simulink subsystem "heat_sink"  (R2020b)
settings: Solver=VariableStepAuto  StartTime=0.0  StopTime=10.0  RelTol=1e-3
model mask{fidelityPARAM=Reduced Order Model, freqPARAM=[-Inf 20], kPARAM=64}
  mask prompts: fidelityPARAM "Choose fidelity:"; freqPARAM "Frequency Range:"; kPARAM "Frequencies retained:"
values from neighbouring files (symbols this model uses):
  h_forced = [  0.0, h_free;  3.0, 50.0;  ]    [heat_sink_defs.m]
  h_free = 9.0    (= 9)    [heat_sink_defs.m]
  normalizedForcedBC = zeros(nDoF,1)    [heat_sink_defs.m]
  normalizedFreeBC = zeros(nDoF,1)    [heat_sink_defs.m]
  Tinf = IC    (= 294)    [heat_sink_defs.m]
  unitCPUHeat = full(F)    [heat_sink_defs.m]
  unitForcedBC = zeros(nDoF,1)    [heat_sink_defs.m]
  unitFreeBC = zeros(nDoF,1)    [heat_sink_defs.m]
  x0 = ones(nDoF,1)*IC    [heat_sink_defs.m]
undefined symbols (not defined in the file or in its folder): Ar, Br, Cr, Dr, sparse, speye, V
settings Model: Creator=jclinton  LastModifiedBy=jclinton
settings DebuggingCC: SFMachineParentedDataDiag=error

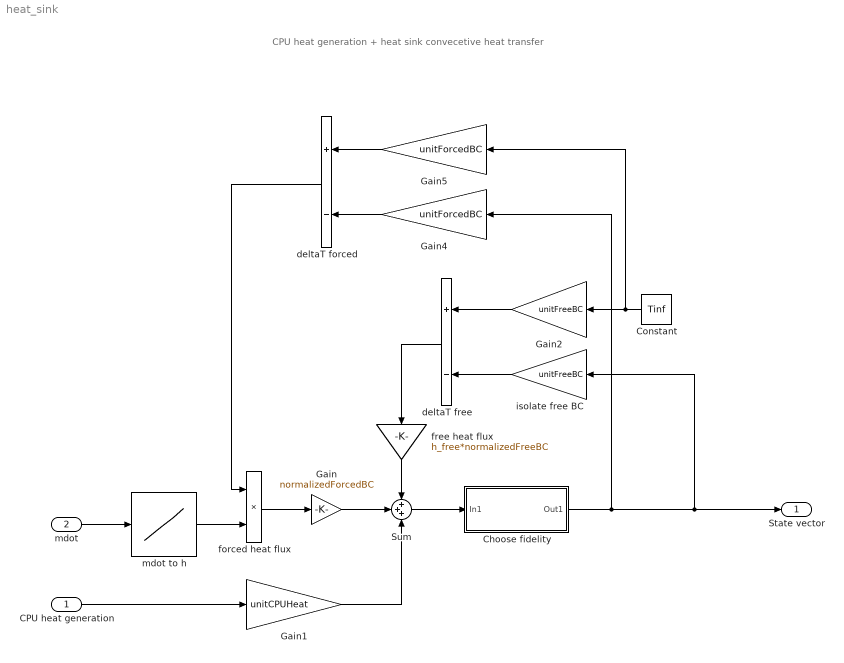
== system heat_sink ==
  note: CPU heat generation + heat sink convecetive heat transfer
  CPU heat generation : Inport  Unit=W
  mdot : Inport  Port=2  Unit=kg/sec
  Choose fidelity : Subsystem  Variant=on  VariantControlMode=label  LabelModeActiveChoice=Choice_2
      mask init:
      | fidelity = get_param(gcs,'fidelityPARAM');
      | vssBlk = gcb;
      | if strcmp(fidelity,'Finite Element Model')
      |     set_param(vssBlk, 'LabelModeActiveChoice', 'Choice_1');
      | else
      |     set_param(vssBlk, 'LabelModeActiveChoice', 'Choice_2');
      |     Q = evalin('base','Q');
      |     K = evalin('base','K');
      |     nDoF = evalin('base','nDoF');
      |     M = evalin('base','M');
      |     freq = str2num(get_param(gcs,'freqPARAM'));
      |     k = str2num(get_param(gcs,'kPARAM'));
      |     [Ar,Br,Cr,Dr,Er,V] = reduceModelOrder(Q+K, ...
      |                                           speye(nDoF,nDoF), ...
      |                                           speye(nDoF,nDoF), ...
      |                                           sparse(nDoF,nDoF), ...
      |                                           M, ...
      |                                           freq,...
      |                                           k);
      | end
      mask DialogControl DescGroupVar Prompt: Choose between FE formulation or a reduced order model
      mask DialogControl DescTextVar Prompt: Different DSS blocks underneath mask chosen depending on desirede fidelity
      mask Display: disp('\partialu/\partialt = \alpha(\Deltau)','texmode','on')
  Constant : Constant  Value=Tinf
  Gain : Gain  Gain=normalizedForcedBC
  Gain1 : Gain  Gain=unitCPUHeat
  Gain2 : Gain  Gain=unitFreeBC
  Gain4 : Gain  Gain=unitForcedBC
  Gain5 : Gain  Gain=unitForcedBC
  Sum : Sum  Inputs=+++
  "deltaT forced " : Sum  Inputs=+-
  deltaT free : Sum  Inputs=+-
  forced heat flux : Product
  free heat flux : Gain  Gain=h_free*normalizedFreeBC
  isolate free BC : Gain  Gain=unitFreeBC
  mdot to h : Lookup_n-D  NumberOfTableDimensions=1  BreakpointsForDimension1=h_forced(:,1)  Table=h_forced(:,2)  InternalRulePriority=Speed  RndMeth=Simplest  InputSameDT=on
  State vector : Outport  Unit=K
  wires:
  mdot/1 -> mdot to h/1
  mdot to h/1 -> forced heat flux/2
  forced heat flux/1 -> Gain/1
  Gain/1 -> Sum/2
  free heat flux/1 -> Sum/1
  deltaT free/1 -> free heat flux/1
  Gain2/1 -> deltaT free/1
  Constant/1 -> Gain5/1, Gain2/1
  isolate free BC/1 -> deltaT free/2
  Gain4/1 -> "deltaT forced "/2
  Gain5/1 -> "deltaT forced "/1
  "deltaT forced "/1 -> forced heat flux/1
  CPU heat generation/1 -> Gain1/1
  Gain1/1 -> Sum/3
  Choose fidelity/1(Out1) -> Gain4/1, State vector/1, isolate free BC/1
  Sum/1 -> Choose fidelity/1(In1)

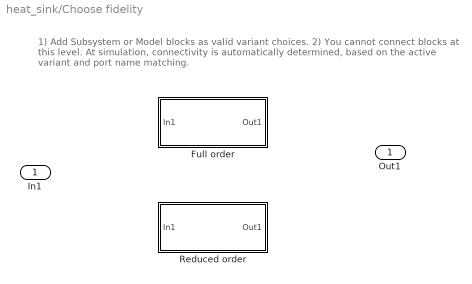
== system heat_sink/Choose fidelity ==
  note: 1) Add Subsystem or Model blocks as valid variant choices.
      | 2) You cannot connect blocks at this level. At simulation, connectivity is automatically
      | determined, based on the active variant and port name matching.
  In1 : Inport
  Full order : Subsystem  VariantControl=Choice_1
  Reduced order : Subsystem  VariantControl=Choice_2
  Out1 : Outport

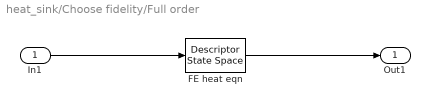
== system heat_sink/Choose fidelity/Full order ==
  In1 : Inport
  FE heat eqn : DescriptorStateSpace  E=M  A=-(Q+K)  B=speye(nDoF,nDoF)  C=speye(nDoF,nDoF)  D=sparse(nDoF,nDoF)  InitialCondition=x0  DirectFeedthrough=False
  Out1 : Outport
  wires:
  FE heat eqn/1 -> Out1/1
  In1/1 -> FE heat eqn/1

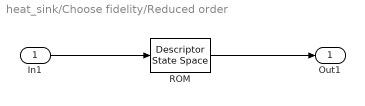
== system heat_sink/Choose fidelity/Reduced order ==
  In1 : Inport
  ROM : DescriptorStateSpace  E=Er  A=-Ar  B=Br  C=Cr  D=Dr  InitialCondition=V'*x0  DirectFeedthrough=False
  Out1 : Outport
  wires:
  ROM/1 -> Out1/1
  In1/1 -> ROM/1
